simulink model "PMSM_Trapezoidal_OpenLoop"  (R2013b)
settings: Solver=ode45  StartTime=0.0  StopTime=8  RelTol=1e-3
undefined symbols (not defined in the file): Plot_PMSM
libraries: powerlib x6
CloseFcn:
  | clear tout
settings Model: Creator=Alex  LastModifiedBy=reynaudp
settings OptimizationCC: ExpressionDepthLimit=2147483647
settings DebuggingCC: UnconnectedLineMsg=none  StateNameClashWarn=warning

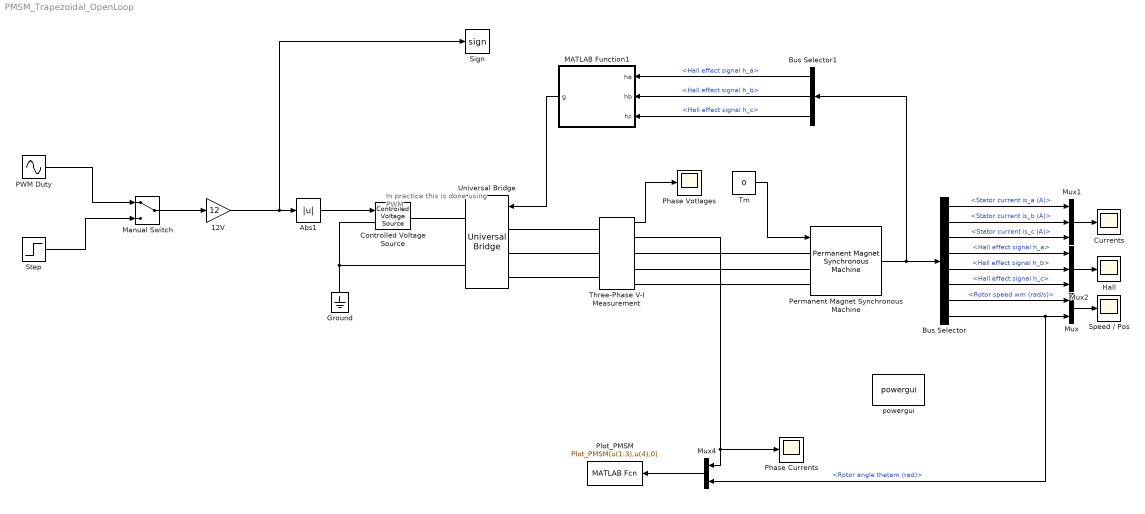
== system PMSM_Trapezoidal_OpenLoop ==
  note: In practice this is done using PWM
  12V : Gain  Gain=12
  Abs1 : Abs
  Bus Selector : BusSelector  OutputSignals=Stator current is_a (A),Stator current is_b (A),Stator current is_c (A),Hall effect signal h_a,Hall effect signal h_b,Hall effect signal h_c,Rotor speed wm (rad/s),Rotor angle thetam (rad)
  Bus Selector1 : BusSelector  OutputSignals=Hall effect signal h_a,Hall effect signal h_b,Hall effect signal h_c
  Controlled Voltage Source : powerlib/Electrical Sources/Controlled Voltage Source  Initialize=on  Source_Type=AC  Amplitude=0  Phase=0  Frequency=0  Measurements=None
  Currents : Scope
      settings: YMin=-1  YMax=1
  Ground : powerlib/Elements/Ground  LConnTagsString=a
  Hall : Scope
      settings: ShowLegends=on  TimeRange=1  YMin=0  YMax=1  SaveName=ScopeData2
  MATLAB Function1 : MATLAB Function  TreatAsAtomicUnit=on
  Manual Switch : ManualSwitch
  Mux : Mux  Inputs=2
  Mux1 : Mux  Inputs=3
  Mux2 : Mux  Inputs=3
  Mux4 : Mux  Inputs=2
  PWM Duty : Sin  Frequency=2*pi*0.1  SampleTime=0
  Permanent Magnet Synchronous Machine : powerlib/Machines/Permanent Magnet Synchronous Machine  NbPhases=3  FluxDistribution=Trapezoidal  RotorType=Round  MechanicalLoad=Torque Tm  PresetModel=No  ShowDetailedParameters=on  Resistance=0.6  Inductance=1.4e-3  dqInductances=[8.5e-3,8.5e-3]  La=0.000835  MachineConstant=Voltage Constant (V_peak L-L / krpm)  Flux=0.0295  VoltageCst=6.1785  TorqueCst=0.059  Flat=120  Mechanical=[1.1e-5,0,1,0.02]  PolePairs=1  InitialConditions=[1,0 0,0]  InitialConditions5ph=[0 0 0 0 0 0]  TsPowergui=0  TsBlock=-1  RefAngle=Aligned with phase A axis (original Park)
  Phase Currents : Scope
      settings: YMin=-7  YMax=7  SaveName=ScopeData4
  Phase Votlages : Scope
      settings: YMin=-1  YMax=13  SaveName=ScopeData3
  Plot_PMSM : MATLABFcn  MATLABFcn=Plot_PMSM(u(1:3),u(4),0)  OutputDimensions=0  SampleTime=1/1000
  Sign : Signum
  Speed / Pos : Scope
      settings: ShowLegends=on  TimeRange=8  YMin=0  YMax=120
  Step : Step  Time=0.1  SampleTime=0
  Three-Phase V-I Measurement : powerlib/Measurements/Three-Phase V-I Measurement  VoltageMeasurement=phase-to-ground  SetLabelV=off  LabelV=Vabc  Vpu=off  VpuLL=off  CurrentMeasurement=yes  SetLabelI=off  LabelI=Iabc  Ipu=off  Pbase=100e6  Vbase=500e3  OutputType=Complex  PhasorSimulation=off  PSBequivalent=0
  Tm : Constant  Value=0
  Universal Bridge : powerlib/Power Electronics/Universal Bridge  Arms=3  SnubberResistance=1e5  SnubberCapacitance=inf  Device=MOSFET / Diodes  Ron=1e-3  Lon=0  ForwardVoltages="[  0  0  ]"  ForwardVoltage=0  GTOparameters=[ 10e-6 , 20e-6 ]  IGBTparameters=[ 1e-6 , 2e-6 ]  Measurements=None  Measurements_2=None  converterType=Rectifier
  powergui : powerlib/powergui  Priority=1  SimulationMode=Discrete  SolverType=Tustin  SampleTime=10e-6  frequency=60  SPID=off  DisableSnubberDevices=off  DisableRonSwitches=off  DisableVfSwitches=off  SwTol=0  Interpol=off  DisplayEquations=off  frequencyindice=0  Pbase=100e6  ErrMax=1e-4  Iterations=50  UnitsV=kV  UnitsW=MW  FunctionMessages=off  echomessages=off  HookPort=off  EnableUseOfTLC=off  x0status=blocks  RestoreLinks=warning  ResistiveCurrentMeasurement=off  Frange=[0:2:500]  Ylog=off  Xlog=on  ShowGrid=off  save=off  variable=ZData  ZoomFFT=off  StartTime=0.0  cycles=1  DisplayStyle=1  fundamental=60  FreqAxis=off  MaxFrequency=1000  frequencyindicesteady=1  RmsSteady=1  display=off  Ts=0  methode=off
  wires:
  Bus Selector/1 -> Mux1/1  "<Stator current is_a (A)>"
  Bus Selector/2 -> Mux1/2  "<Stator current is_b (A)>"
  Bus Selector/3 -> Mux1/3  "<Stator current is_c (A)>"
  Bus Selector/8 -> Mux4/2, Mux/2  "<Rotor angle thetam (rad)>"
  Mux1/1 -> Currents/1
  Tm/1 -> Permanent Magnet Synchronous Machine/1
  Permanent Magnet Synchronous Machine/1 -> Bus Selector1/1, Bus Selector/1
  Bus Selector/7 -> Mux/1  "<Rotor speed wm (rad/s)>"
  Bus Selector/4 -> Mux2/1  "<Hall effect signal h_a>"
  Bus Selector/5 -> Mux2/2  "<Hall effect signal h_b>"
  Bus Selector/6 -> Mux2/3  "<Hall effect signal h_c>"
  Mux2/1 -> Hall/1
  Three-Phase V-I Measurement/1 -> Phase Votlages/1
  Mux/1 -> Speed / Pos/1
  Abs1/1 -> Controlled Voltage Source/1
  12V/1 -> Sign/1, Abs1/1
  Mux4/1 -> Plot_PMSM/1
  Manual Switch/1 -> 12V/1
  PWM Duty/1 -> Manual Switch/1
  Step/1 -> Manual Switch/2
  Three-Phase V-I Measurement/2 -> Phase Currents/1, Mux4/1
  MATLAB Function1/1(g) -> Universal Bridge/1
  Bus Selector1/1 -> MATLAB Function1/1(ha)  "<Hall effect signal h_a>"
  Bus Selector1/2 -> MATLAB Function1/2(hb)  "<Hall effect signal h_b>"
  Bus Selector1/3 -> MATLAB Function1/3(hc)  "<Hall effect signal h_c>"
  connections:
  Three-Phase V-I Measurement/RConn1 -- Permanent Magnet Synchronous Machine/LConn1
  Three-Phase V-I Measurement/RConn2 -- Permanent Magnet Synchronous Machine/LConn2
  Three-Phase V-I Measurement/RConn3 -- Permanent Magnet Synchronous Machine/LConn3
  Controlled Voltage Source/LConn1 -- Ground/LConn1 -- Universal Bridge/RConn2
  Controlled Voltage Source/RConn1 -- Universal Bridge/RConn1
  Universal Bridge/LConn1 -- Three-Phase V-I Measurement/LConn1
  Universal Bridge/LConn2 -- Three-Phase V-I Measurement/LConn2
  Universal Bridge/LConn3 -- Three-Phase V-I Measurement/LConn3

== matlab function PMSM_Trapezoidal_OpenLoop/MATLAB Function1 ==
  data: ha input; hb input; hc input; g output
function g=Hall_State(ha,hb,hc)

ab = ha & ~hb & hc;
ba = ~ha & hb & ~hc;
ac = ha & ~hb & ~hc;
ca = ~ha & hb & hc;
bc = ha & hb & ~hc;
cb = ~ha & ~hb & hc;


g = [(ab | ac),(ba | ca), (ba | bc), (ab |cb), (ca | cb), (ac | bc)];
